simulink model "fullcircuit"  (R2020a)
settings: Solver=VariableStepAuto  StartTime=0.0  StopTime=5  RelTol=1e-3
undefined symbols (not defined in the file): Acid, Down, Lead, Up
libraries: powerlib x27, eeGeneralControl x4, electricdrivelib x1, eePwmGenerator x1
settings Model: Creator=Asus  LastModifiedBy=asus
settings DataIOCC: ReturnWorkspaceOutputs=off
settings DebuggingCC: ArithmeticOperatorsInVariantConditions=warning
settings SFSimCC: CustomCodeUndefinedFunction=UseInterfaceOnly

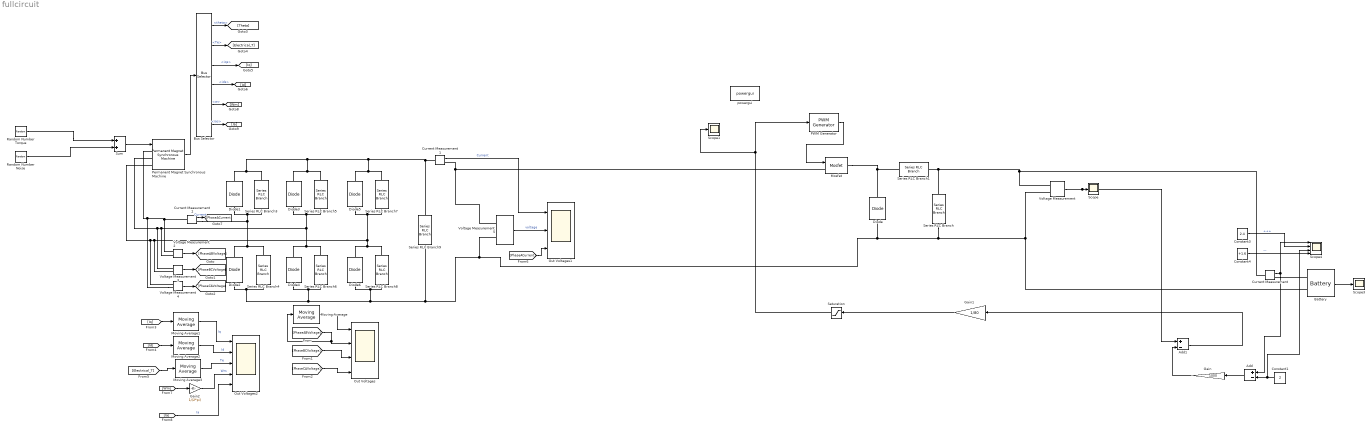
== system fullcircuit ==
  Add : Sum  Inputs=+-
  Add1 : Sum  Inputs=+-
  Battery : electricdrivelib/Extra Sources/Battery  BatType=Lead-Acid  ShowTempParam=off  ThermalPreset=no  ShowAgeParam=off  NomV=24  NomQ=13  SOC=50  Batt_Tr=0.000001  PresetModel=on  MaxQ=13.5417  MinV=18  FullV=26.1316  Dis_rate=2.6  R=0.018462  Normal_OP=4.0336  expZone="[24.4342    0.0433333]"  current=[6.5 13 32.5]  Units=Time  Tci=20  NomT=20  T2=-30  MaxQ2=4.8  FullV2=7.1  Normal_OP2=5.655  expZone2="[6.58           1]"  Rca=0.6  ti=2000  Dp=0  Neq0=0  Tsim=1e6  Ta1=25  Qeol=5.4*0.9  Reol=0.013333*1.2  Char_age=[2.3478, 3]  Dis_age=[2.3478, 10]  N1=1500  N2=10500  N3=1000  N4=1400  Ta2=45  N5=950
  Bus Selector : BusSelector  OutputSignals=theta,Te,iqs,ids,w,ias
  Constant1 : Constant  Value=2
  Constant3 : Constant  Value=2.4
  Constant4 : Constant  Value=+1.6
  Current Measurement : powerlib/Measurements/Current Measurement  PhasorSimulation=off  OutputType=Complex  PSBequivalent=0
  Current Measurement1 : powerlib/Measurements/Current Measurement  PhasorSimulation=off  OutputType=Complex  PSBequivalent=0
  Current Measurement2 : powerlib/Measurements/Current Measurement  PhasorSimulation=off  OutputType=Complex  PSBequivalent=0
  Diode : powerlib/Power Electronics/Diode  Ron=0.001  Lon=0  Vf=0.8  IC=0  UseSnubber=0  Rs=500  Cs=250e-9  Measurements=off
  Diode{1..6} (6 alike) : powerlib/Power Electronics/Diode  Ron=0.001  Lon=0  Vf=0  IC=0  UseSnubber=0  Rs=0  Cs=0  Measurements=off
  Gain : Gain  Gain=1000
  Gain1 : Gain  Gain=1/80
  Gain2 : Gain  Gain=1/(2*pi)
  Mosfet : powerlib/Power Electronics/Mosfet  Ron=0.1  Lon=0  Rd=0.01  Vfd=0  IC=0  Rs=1e5  Cs=inf  Measurements=off
  Moving Average : eeGeneralControl/Moving Average  VariantControl=Variant1  LabelModeActiveChoice=Discrete  f=1000  x0=0  Ts=10e-6
      settings: SourceProductBaseCode=PS
  Moving Average1 : eeGeneralControl/Moving Average  VariantControl=Variant1  LabelModeActiveChoice=Discrete  f=100  x0=0  Ts=1e-5
      settings: SourceProductBaseCode=PS
  Moving Average2 : eeGeneralControl/Moving Average  VariantControl=Variant1  LabelModeActiveChoice=Discrete  f=100  x0=0  Ts=1e-5
      settings: SourceProductBaseCode=PS
  Moving Average3 : eeGeneralControl/Moving Average  VariantControl=Variant1  LabelModeActiveChoice=Discrete  f=100  x0=0  Ts=1e-5
      settings: SourceProductBaseCode=PS
  Out Voltages : Scope  NumInputPorts=4
  Out Voltages1 : Scope  NumInputPorts=3
  Out Voltages2 : Scope  NumInputPorts=5
  PWM Generator : eePwmGenerator/PWM Generator  CarrCount=Up-Down  Tper=1e-4  Ts=5e-6
  Permanent Magnet Synchronous Machine : powerlib/Machines/Permanent Magnet Synchronous Machine  NbPhases=3  FluxDistribution=Sinusoidal  RotorType=Round  MechanicalLoad=Torque Tm  PresetModel=No  ShowDetailedParameters=on  MeasurementBus=on  Resistance=10.58  Inductance=8.5e-3  dqInductances=[8.5e-3,8.5e-3]  La=16.7e-3  MachineConstant=Voltage Constant (V_peak L-L / krpm)  Flux=0.60646  VoltageCst=110  TorqueCst=0.90969  Flat=120  Mechanical=[0.00027 0.005024 1 0]  PolePairs=4  InitialConditions=[100,0, 0,0]  InitialConditions5ph=[0 0 0 0 0 0]  RefAngle=90 degrees behind phase A axis (modified Park)  IterativeDiscreteModel=Trapezoidal non iterative  TsBlock=-1  TsPowergui=0
  Random Number Noise : RandomNumber  Variance=0.1  SampleTime=1e-3
  Random Number Torque : RandomNumber  Mean=-1.6  Variance=0.05  SampleTime=0.1
  Saturation : Saturate  UpperLimit=1  LowerLimit=0  ZeroCross=off
  Scope : Scope
  Scope1 : Scope
  Scope3 : Scope
  Scope4 : Scope  NumInputPorts=4
  Series RLC Branch : powerlib/Elements/Series RLC Branch  LConnTagsString=__new0  RConnTagsString=__new0  BranchType=RC  Resistance=0.2  Inductance=1e-9  SetiL0=off  InitialCurrent=0  Capacitance=1.63e-6  Setx0=on  InitialVoltage=24.1  Measurements=None
  Series RLC Branch1 : powerlib/Elements/Series RLC Branch  LConnTagsString=__new0  RConnTagsString=__new0  BranchType=L  Resistance=1  Inductance=0.012  SetiL0=off  InitialCurrent=0  Capacitance=1e-6  Setx0=off  InitialVoltage=0  Measurements=None
  Series RLC Branch{3..8} (6 alike) : powerlib/Elements/Series RLC Branch  LConnTagsString=__new0  RConnTagsString=__new0  BranchType=R  Resistance=1e6  Inductance=1e-3  SetiL0=off  InitialCurrent=0  Capacitance=1e-6  Setx0=off  InitialVoltage=0  Measurements=None
  Series RLC Branch9 : powerlib/Elements/Series RLC Branch  LConnTagsString=__new0  RConnTagsString=__new0  BranchType=C  Resistance=1e6  Inductance=1e-3  SetiL0=off  InitialCurrent=0  Capacitance=470e-6  Setx0=on  InitialVoltage=225  Measurements=None
  Sum : Sum  Inputs=+|+
  Voltage Measurement{,2..5} (5 alike) : powerlib/Measurements/Voltage Measurement  PhasorSimulation=off  OutputType=Complex  PSBequivalent=0
  powergui : powerlib/powergui  Priority=1  SimulationMode=Continuous  SampleTime=50e-6  frequency=60  Iterations=50  frequencyindice=0  Pbase=100e6  ErrMax=1e-4  UnitsV=kV  UnitsW=MW  buscounter=0  FunctionMessages=off  echomessages=off  EnableUseOfTLC=off  CurrentSourceSwitches=off  DisableSnubberDevices=off  DisableRonSwitches=off  DisableVfSwitches=off  DisplayEquations=off  AutomaticDiscreteSolvers=off  SolverType=Tustin/Backward Euler (TBE)  Interpol=off  ExternalGateDelay=off  methode=off  Ts=100  x0status=blocks  SPID=on  SwTol=0  HookPort=off  NonlinearTolerance=1e-4  nMaxIteration=100  ContinueOnMaxIteration=off  RestoreLinks=warning  ResistiveCurrentMeasurement=off  Frange=[0:2:500]  Ylog=off  Xlog=on  ShowGrid=off  save=off  variable=ZData  structure=0  ZoomFFT=off  StartTime=0.0  cycles=1  DisplayStyle=1  fundamental=60  FreqAxis=off  MaxFrequency=1000  frequencyindicesteady=1  RmsSteady=1  display=off
  wires:
  PWM Generator/1 -> Mosfet/1
  Voltage Measurement/1 -> Add1/1, Scope/1
  Constant3/1 -> Scope4/2  "+++"
  Gain1/1 -> Saturation/1
  Gain/1 -> Add1/2
  Current Measurement/1 -> Scope4/1, Add/1
  Add/1 -> Gain/1
  Constant1/1 -> Scope4/3, Add/2
  Add1/1 -> Gain1/1
  Constant4/1 -> Scope4/4  "---"
  Battery/1 -> Scope3/1
  Moving Average1/1 -> Out Voltages2/1  "Iq"
  Bus Selector/4 -> [Id]  "<ids>"
  [Ia] -> Out Voltages2/5  "Ia"
  Bus Selector/6 -> [Ia]  "<ias>"
  Bus Selector/5 -> [Wm]  "<w>"
  [Wm] -> Gain2/1
  [PhaseACurrent] -> Out Voltages1/3
  [Electrical_T] -> Moving Average3/1
  Current Measurement2/1 -> [PhaseACurrent]  "Current"
  Moving Average2/1 -> Out Voltages2/2  "Id"
  [PhaseCAVoltage] -> Out Voltages/4
  Bus Selector/3 -> [Iq]  "<iqs>"
  [Id] -> Moving Average2/1
  [Iq] -> Moving Average1/1
  Permanent Magnet Synchronous Machine/1 -> Bus Selector/1
  [PhaseABVoltage] -> Moving Average/1, Out Voltages/2
  Voltage Measurement3/1 -> [PhaseBCVoltage]
  Voltage Measurement2/1 -> [PhaseABVoltage]
  Random Number Torque/1 -> Sum/1
  Bus Selector/1 -> [Theta]  "<theta>"
  Current Measurement1/1 -> Out Voltages1/1  "Current"
  Voltage Measurement4/1 -> [PhaseCAVoltage]
  Random Number Noise/1 -> Sum/2
  Voltage Measurement5/1 -> Out Voltages1/2  "voltage"
  Gain2/1 -> Out Voltages2/4  "Wm"
  Bus Selector/2 -> [Electrical_T]  "<Te>"
  Moving Average3/1 -> Out Voltages2/3  "Te"
  Moving Average/1 -> Out Voltages/1
  [PhaseBCVoltage] -> Out Voltages/3
  Sum/1 -> Permanent Magnet Synchronous Machine/1
  Saturation/1 -> Scope1/1, PWM Generator/1
  connections:
  Current Measurement1/RConn1 -- Voltage Measurement5/LConn1 -- Mosfet/LConn1
  Mosfet/RConn1 -- Series RLC Branch1/LConn1 -- Diode/RConn1
  Diode4/LConn1 -- Diode2/LConn1 -- Series RLC Branch4/RConn1 -- Diode6/LConn1 -- Series RLC Branch8/RConn1 -- Series RLC Branch9/RConn1 -- Voltage Measurement/LConn2 -- Battery/LConn2 -- Series RLC Branch/RConn1 -- Diode/LConn1 -- Voltage Measurement5/LConn2 -- Series RLC Branch6/RConn1
  Voltage Measurement/LConn1 -- Current Measurement/LConn1 -- Series RLC Branch/LConn1 -- Series RLC Branch1/RConn1
  Current Measurement/RConn1 -- Battery/LConn1
  Diode5/LConn1 -- Series RLC Branch7/RConn1 -- Diode6/RConn1 -- Series RLC Branch8/LConn1 -- Permanent Magnet Synchronous Machine/LConn3 -- Voltage Measurement4/LConn1 -- Voltage Measurement3/LConn2
  Voltage Measurement4/LConn2 -- Current Measurement2/LConn1 -- Voltage Measurement2/LConn1 -- Permanent Magnet Synchronous Machine/LConn1
  Series RLC Branch5/RConn1 -- Series RLC Branch6/LConn1 -- Diode4/RConn1 -- Permanent Magnet Synchronous Machine/LConn2 -- Voltage Measurement3/LConn1 -- Voltage Measurement2/LConn2 -- Diode3/LConn1
  Diode3/RConn1 -- Diode1/RConn1 -- Series RLC Branch3/LConn1 -- Series RLC Branch9/LConn1 -- Current Measurement1/LConn1 -- Series RLC Branch7/LConn1 -- Diode5/RConn1 -- Series RLC Branch5/LConn1
  Series RLC Branch3/RConn1 -- Diode1/LConn1 -- Current Measurement2/RConn1 -- Series RLC Branch4/LConn1 -- Diode2/RConn1
